simulink model "quadrotor"  (R2018b)
settings: Solver=VariableStepAuto  StartTime=0.0  StopTime=30  MaxStep=1e-1  RelTol=1e-3  EnableMultiTasking=on
values from neighbouring files (symbols this model uses):
  b = 0.6    [setup.m]
  d = 0.3    [setup.m]
  g = 9.81    [setup.m]
  m = 1    [setup.m]
  M2B_INV = inv(M2B)    [setup.m]
  P_q = 6    [setup.m]
  P_w = 1    [setup.m]
undefined symbols (not defined in the file or in its folder): X, Y, Z
libraries: nesl_utility x18, sm_lib x17
settings Model: Creator=valeriiche  LastModifiedBy=valeriiche
settings DataIOCC: LimitDataPoints=on
settings OptimizationCC: LifeSpan=inf
settings DebuggingCC: AllowSymbolicDim=off  SFUnexpectedBacktrackingDiag=warning  SFNoUnconditionalDefaultTransitionDiag=warning  SFExecutionAtInitializationDiag=none
settings SFSimCC: SimUseLocalCustomCode=off
settings RTWCC: RTWUseLocalCustomCode=off
settings CodeAppCC: StateflowObjectComments=on
settings GRTTargetCC: TargetLangStandard=C89/C90 (ANSI)  GeneratePreprocessorConditionals=Disable all
settings ConfigComp: CovMetricSettings=dw  CovHtmlReporting=on  CovSaveCumulativeToWorkspaceVar=on  CovSaveSingleToWorkspaceVar=on  CovExternalEMLEnable=off  CovSFcnEnable=off
settings SimscapeCC: SimscapeNominalValues="[{\"value\":\"10\",\"unit\":\"V\"},{\"value\":\"1\",\"unit\":\"A\"},{\"value\":\"10\",\"unit\":\"N*m\"},{\"value\":\"10\",\"unit\":\"bar\"},{\"value\":\"100\",\"unit\":\"kJ/kg\"},{\"value\":\"1\",\"unit\":\"kW\"},{\"value\":\"300\",\"unit\":\"K\"},{\"value\":\"100\",\"unit\":\"cm^3/s\"},{\"value\":\"1\",\"unit\":\"kN\"},{\"value\":\"1\",\"unit\":\"g/cm^3\"},{\"value\":\"1\",\"unit\":\"l\"},{\"value\":\"1\",\"unit\":\"cm^2\"},{\"value\":\"60\",\"unit\":\"Hz\"}]"  SimscapeLogType=all  SimscapeLogDataHistory=10000
settings ConfigurationSet: Description=SimMechanics 2G

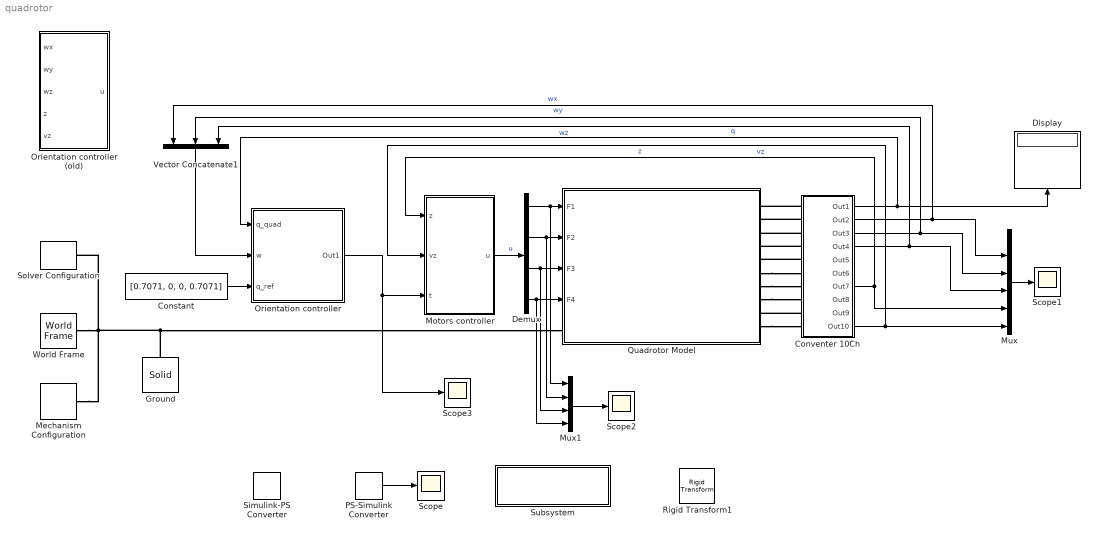
== system quadrotor ==
  Constant : Constant  Value=[0.7071, 0, 0, 0.7071]
  Conventer 10Ch : Subsystem
  Demux : Demux
  Display : Display
  Ground : sm_lib/Body Elements/Solid  InertiaType=CalculateFromGeometry  Mass=1  MassUnits=kg  CenterOfMass=[0 0 0]  CenterOfMassUnits=m  MomentsOfInertia=[1 1 1]  MomentsOfInertiaUnits=kg*m^2  ProductsOfInertia=[0 0 0]  ProductsOfInertiaUnits=kg*m^2  BasedOnType=Density  Density=1000  DensityUnits=kg/m^3  DoExposeReferenceFrame=on  SerializedFrames=<Frames/>  GraphicType=FromGeometry  MarkerShape=Sphere  MarkerSize=10  GraphicVisPropType=SimpleVisualProperties  GraphicDiffuseColor=[0.5 0.5 0.5]  GraphicSpecularColor=[0.5 0.5 0.5 1.0]  GraphicAmbientColor=[0.15 0.15 0.15 1.0]  GraphicEmissiveColor=[0.0 0.0 0.0 1.0]  GraphicShininess=75  GraphicOpacity=1.0  GeometryShape=Brick  RectangleSize=[1 1]  RectangleSizeUnits=m  BrickDimensions=[5 5 0.1]  BrickDimensionUnits=m  CylinderRadius=1  CylinderRadiusUnits=m  CylinderLength=1  CylinderLengthUnits=m  SphereRadius=1  SphereRadiusUnits=m  EllipsoidRadii=[1 1 1]  EllipsoidRadiiUnits=m  ExtrusionCrossSection=[1 1; -1 1; -1 -1; 1 -1]  ExtrusionCrossSectionUnits=m  ExtrusionLength=1  ExtrusionLengthUnits=m  PolygonNumSides=3  PolygonOuterRadius=1  PolygonOuterRadiusUnits=m  ExtGeomFileType=STEP  ExtGeomFileUnits=m  RevolutionCrossSection=[1 1; 1 -1; 2 -1; 2 1]  RevolutionCrossSectionUnits=m  RevolutionExtent=Full  RevolutionAngle=180  RevolutionAngleUnits=deg
  Mechanism Configuration : sm_lib/Utilities/Mechanism Configuration  UniformGravity=Constant  GravityVector=[0 0 -9.80665]  GravityUnits=m/s^2  LinearizationDelta=0.001
  Motors controller : Subsystem
  Mux : Mux  Inputs=6
  Mux1 : Mux
  Orientation controller : Subsystem
  Orientation controller (old) : Subsystem
  PS-Simulink Converter : nesl_utility/PS-Simulink Converter  PhysicalDomain=network_engine_domain  SubClassName=ps_output  LeftPortType=input  RightPortType=output  PseudoPeriodic=off  Frequencies=[]  Unit=1  AffineConversion=off
  Quadrotor Model : Subsystem
  Rigid Transform1 : sm_lib/Frames and Transforms/Rigid Transform  TranslationMethod=None  TranslationStandardOffset=0  TranslationLengthUnit=m  TranslationStandardAxis=+Z  TranslationCartesianOffset=[0 0 0]  TranslationROffset=0  TranslationROffsetUnits=m  TranslationZOffset=0  TranslationZOffsetUnits=m  TranslationThetaOffset=0  TranslationThetaOffsetUnits=deg  RotationMethod=None  RotationAngleUnits=deg  RotationStandardAxis=+Z  RotationAngle=0.0  RotationArbitraryAxis=[0 0 1]  FollAlignAxisA=+X  BaseAlignAxisA=+Y  FollAlignAxisB=+Y  BaseAlignAxisB=+Z  RotationSequenceAxes=FollowerAxes  RotationSequence=XYX  RotationSequenceAngles=[0 0 0]  RotationSequenceAnglesUnits=deg  RotationMatrix=[1 0 0; 0 1 0; 0 0 1]
  Scope{,1..3} (4 alike) : Scope
  Simulink-PS Converter : nesl_utility/Simulink-PS Converter  PhysicalDomain=network_engine_domain  SubClassName=ps_input  LeftPortType=input  RightPortType=output  PseudoPeriodic=off  Frequencies=[]  NoiseDistribution=none  NoiseParameters=[]  Unit=1  AffineConversion=off  FilteringAndDerivatives=zero  SimscapeFilterOrder=1  InputFilterTimeConstant=0.001  UdotUserProvided=1
  Solver Configuration : nesl_utility/Solver Configuration  PhysicalDomain=network_engine_domain  SubClassName=solver  LeftPortType=input  RightPortType=generic  Tones=[]  Harmonics=[]  SimulateNoise=off  Profile=off  UseLocalSampling=off  EnableSwitchedLinearOptims=on  FrequencyDomain=off  UseCCode=off  RelTol=0.001  AbsTol=1e-06  MinStep=1e-09  ToWorkspace=off  RevertToSquareIcSolve=off  NumHomotopyIterations=100  PhasorMode=off  PhasorModeNumHarmonics=1  DoDC=off  ResidualTolerance=1e-09  UseLocalSolver=off  LocalSolverChoice=NE_BACKWARD_EULER_ADVANCER  LocalSolverSampleTime=0.001  DoFixedCost=off  MaxNonlinIter=3  MaxModeIter=2  LinearAlgebra=Sparse  EquationFormulation=NE_TIME_EF  DelaysMemoryBudget=1024  AutomaticFiltering=on  FilteringTimeConstant=0.001  PartitionStorageMethod=AS_NEEDED  PartitionMemoryBudget=1024
  Subsystem : Subsystem
      settings: OpenFcn=open_system('sm_lib')
      mask Display: disp(sprintf('Open Simscape Multibody\nLibrary'));
  Vector Concatenate1 : Concatenate  NumInputs=3
  World Frame : sm_lib/Frames and Transforms/World Frame
  wires:
  PS-Simulink Converter/1 -> Scope/1
  Mux/1 -> Scope1/1
  Conventer 10Ch/3(Out3) -> Mux/3, Vector Concatenate1/2  "wy"
  Conventer 10Ch/7(Out7) -> Mux/5, Motors controller/1(z)  "z"
  Conventer 10Ch/10(Out10) -> Mux/6, Motors controller/2(vz)  "vz"
  Conventer 10Ch/4(Out4) -> Mux/4, Vector Concatenate1/3  "wz"
  Conventer 10Ch/2(Out2) -> Mux/2, Vector Concatenate1/1  "wx"
  Demux/1 -> Mux1/1, Quadrotor Model/1(F1)
  Demux/2 -> Mux1/2, Quadrotor Model/2(F2)
  Conventer 10Ch/1(Out1) -> Orientation controller/1(q_quad), Display/1  "q"
  Motors controller/1(u) -> Demux/1  "u"
  Orientation controller/1(Out1) -> Scope3/1, Motors controller/3(t)
  Vector Concatenate1/1 -> Orientation controller/2(w)
  Constant/1 -> Orientation controller/3(q_ref)
  Mux1/1 -> Scope2/1
  Demux/3 -> Mux1/3, Quadrotor Model/3(F3)
  Demux/4 -> Mux1/4, Quadrotor Model/4(F4)
  connections:
  Ground/RConn1 -- Quadrotor Model/LConn1 -- Solver Configuration/RConn1 -- Mechanism Configuration/RConn1 -- World Frame/RConn1
  Conventer 10Ch/LConn1 -- Quadrotor Model/RConn1
  Conventer 10Ch/LConn2 -- Quadrotor Model/RConn2
  Conventer 10Ch/LConn3 -- Quadrotor Model/RConn3
  Conventer 10Ch/LConn4 -- Quadrotor Model/RConn4
  Conventer 10Ch/LConn5 -- Quadrotor Model/RConn5
  Quadrotor Model/RConn6 -- Conventer 10Ch/LConn6
  Quadrotor Model/RConn7 -- Conventer 10Ch/LConn7
  Quadrotor Model/RConn8 -- Conventer 10Ch/LConn8
  Conventer 10Ch/LConn9 -- Quadrotor Model/RConn9
  Quadrotor Model/RConn10 -- Conventer 10Ch/LConn10

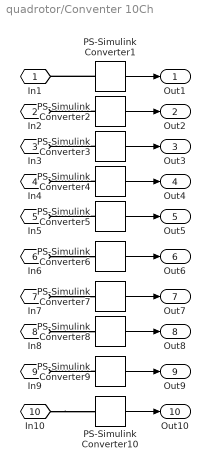
== system quadrotor/Conventer 10Ch ==
  PS-Simulink Converter{1..10} (10 alike) : nesl_utility/PS-Simulink Converter  PhysicalDomain=network_engine_domain  SubClassName=ps_output  LeftPortType=input  RightPortType=output  PseudoPeriodic=off  Frequencies=[]  Unit=1  AffineConversion=off
  In1 : PMIOPort  Side=Left
  In2 : PMIOPort  Port=2  Side=Left
  In3 : PMIOPort  Port=3  Side=Left
  In4 : PMIOPort  Port=4  Side=Left
  In5 : PMIOPort  Port=5  Side=Left
  In6 : PMIOPort  Port=6  Side=Left
  In7 : PMIOPort  Port=7  Side=Left
  In8 : PMIOPort  Port=8  Side=Left
  In9 : PMIOPort  Port=9  Side=Left
  In10 : PMIOPort  Port=10  Side=Left
  Out1 : Outport
  Out2 : Outport  Port=2
  Out3 : Outport  Port=3
  Out4 : Outport  Port=4
  Out5 : Outport  Port=5
  Out6 : Outport  Port=6
  Out7 : Outport  Port=7
  Out8 : Outport  Port=8
  Out9 : Outport  Port=9
  Out10 : Outport  Port=10
  wires:
  PS-Simulink Converter7/1 -> Out7/1
  PS-Simulink Converter4/1 -> Out4/1
  PS-Simulink Converter6/1 -> Out6/1
  PS-Simulink Converter8/1 -> Out8/1
  PS-Simulink Converter5/1 -> Out5/1
  PS-Simulink Converter9/1 -> Out9/1
  PS-Simulink Converter10/1 -> Out10/1
  PS-Simulink Converter3/1 -> Out3/1
  PS-Simulink Converter1/1 -> Out1/1
  PS-Simulink Converter2/1 -> Out2/1
  connections:
  In7/RConn1 -- PS-Simulink Converter7/LConn1
  PS-Simulink Converter1/LConn1 -- In1/RConn1
  PS-Simulink Converter3/LConn1 -- In3/RConn1
  In10/RConn1 -- PS-Simulink Converter10/LConn1
  PS-Simulink Converter2/LConn1 -- In2/RConn1
  In6/RConn1 -- PS-Simulink Converter6/LConn1
  PS-Simulink Converter5/LConn1 -- In5/RConn1
  PS-Simulink Converter4/LConn1 -- In4/RConn1
  In8/RConn1 -- PS-Simulink Converter8/LConn1
  PS-Simulink Converter9/LConn1 -- In9/RConn1

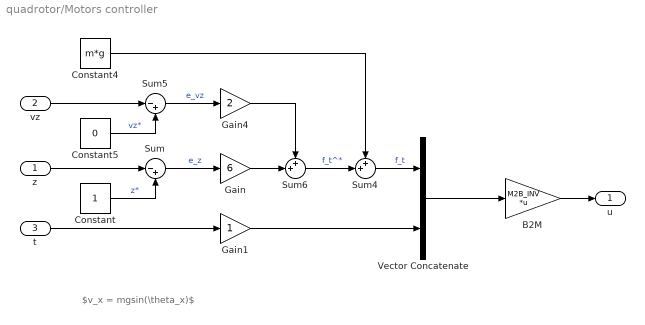
== system quadrotor/Motors controller ==
  note: $v_x = mgsin(\theta_x)$
  z : Inport
  vz : Inport  Port=2
  t : Inport  Port=3
  B2M : Gain  Gain=M2B_INV  Multiplication=Matrix(K*u) (u vector)
  Constant : Constant
  Constant4 : Constant  Value=m*g
  Constant5 : Constant  Value=0
  Gain : Gain  Gain=6
  Gain1 : Gain
  Gain4 : Gain  Gain=2
  Sum : Sum  Inputs=|-+
  Sum4 : Sum  Inputs=++|
  Sum5 : Sum  Inputs=|-+
  Sum6 : Sum  Inputs=++|
  Vector Concatenate : Concatenate
  u : Outport
  wires:
  Sum5/1 -> Gain4/1  "e_vz"
  B2M/1 -> u/1
  Gain/1 -> Sum6/2
  Gain4/1 -> Sum6/1
  z/1 -> Sum/1
  Sum4/1 -> Vector Concatenate/1  "f_t"
  Sum6/1 -> Sum4/2  "f_t^*"
  t/1 -> Gain1/1
  Constant5/1 -> Sum5/2  "vz*"
  Sum/1 -> Gain/1  "e_z"
  Vector Concatenate/1 -> B2M/1
  Gain1/1 -> Vector Concatenate/2
  Constant/1 -> Sum/2  "z*"
  Constant4/1 -> Sum4/1
  vz/1 -> Sum5/1

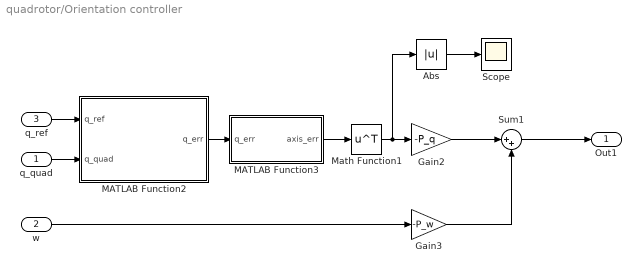
== system quadrotor/Orientation controller ==
  q_quad : Inport
  w : Inport  Port=2
  q_ref : Inport  Port=3
  Abs : Abs
  Gain2 : Gain  Gain=-P_q
  Gain3 : Gain  Gain=-P_w
  MATLAB Function2 : MATLAB Function  TreatAsAtomicUnit=on
  MATLAB Function3 : MATLAB Function  TreatAsAtomicUnit=on
  Math Function1 : Math  Operator=transpose  SaturateOnIntegerOverflow=on
  Scope : Scope
  Sum1 : Sum  Inputs=|++
  Out1 : Outport
  wires:
  Sum1/1 -> Out1/1
  Math Function1/1 -> Abs/1, Gain2/1
  MATLAB Function2/1(q_err) -> MATLAB Function3/1(q_err)
  Gain2/1 -> Sum1/1
  MATLAB Function3/1(axis_err) -> Math Function1/1
  Gain3/1 -> Sum1/2
  q_quad/1 -> MATLAB Function2/2(q_quad)
  q_ref/1 -> MATLAB Function2/1(q_ref)
  w/1 -> Gain3/1
  Abs/1 -> Scope/1

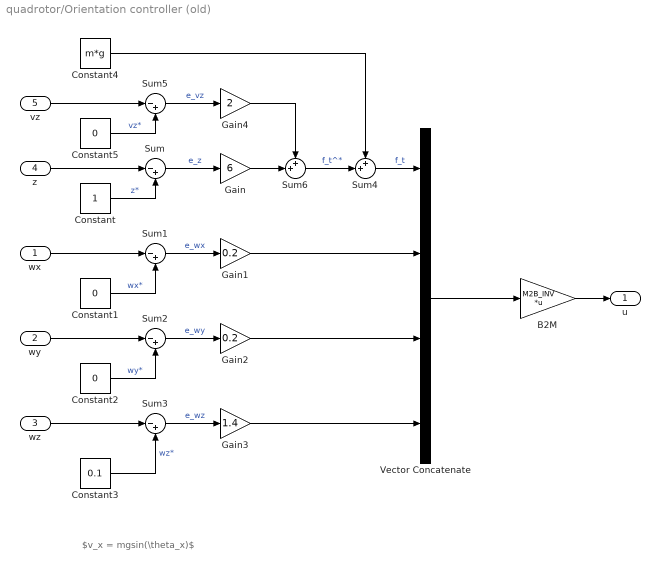
== system quadrotor/Orientation controller (old) ==
  note: $v_x = mgsin(\theta_x)$
  wx : Inport
  wy : Inport  Port=2
  wz : Inport  Port=3
  z : Inport  Port=4
  vz : Inport  Port=5
  B2M : Gain  Gain=M2B_INV  Multiplication=Matrix(K*u) (u vector)
  Constant : Constant
  Constant1 : Constant  Value=0
  Constant2 : Constant  Value=0
  Constant3 : Constant  Value=0.1
  Constant4 : Constant  Value=m*g
  Constant5 : Constant  Value=0
  Gain : Gain  Gain=6
  Gain1 : Gain  Gain=0.2
  Gain2 : Gain  Gain=0.2
  Gain3 : Gain  Gain=1.4
  Gain4 : Gain  Gain=2
  Sum{,1..3,5} (5 alike) : Sum  Inputs=|-+
  Sum4 : Sum  Inputs=++|
  Sum6 : Sum  Inputs=++|
  Vector Concatenate : Concatenate  NumInputs=4
  u : Outport
  wires:
  vz/1 -> Sum5/1
  Constant3/1 -> Sum3/2  "wz*"
  wx/1 -> Sum1/1
  Constant4/1 -> Sum4/1
  Constant/1 -> Sum/2  "z*"
  Sum3/1 -> Gain3/1  "e_wz"
  Gain1/1 -> Vector Concatenate/2
  Vector Concatenate/1 -> B2M/1
  Gain3/1 -> Vector Concatenate/4
  Sum/1 -> Gain/1  "e_z"
  wy/1 -> Sum2/1
  Constant2/1 -> Sum2/2  "wy*"
  Constant1/1 -> Sum1/2  "wx*"
  Sum2/1 -> Gain2/1  "e_wy"
  Constant5/1 -> Sum5/2  "vz*"
  Sum1/1 -> Gain1/1  "e_wx"
  wz/1 -> Sum3/1
  Sum6/1 -> Sum4/2  "f_t^*"
  Sum4/1 -> Vector Concatenate/1  "f_t"
  z/1 -> Sum/1
  Gain4/1 -> Sum6/1
  Gain2/1 -> Vector Concatenate/3
  Gain/1 -> Sum6/2
  B2M/1 -> u/1
  Sum5/1 -> Gain4/1  "e_vz"

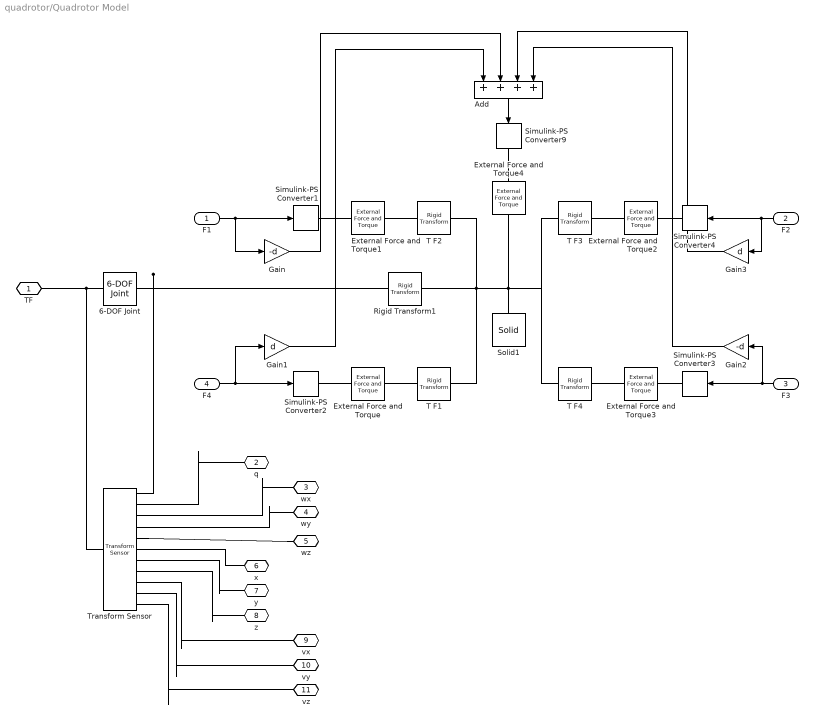
== system quadrotor/Quadrotor Model ==
  F1 : Inport
  F2 : Inport  Port=2
  F3 : Inport  Port=3
  F4 : Inport  Port=4
  6-DOF Joint : sm_lib/Joints/6-DOF Joint  SenseConstraintForce=off  SenseConstraintForceX=off  SenseConstraintForceY=off  SenseConstraintForceZ=off  SenseConstraintTorque=off  SenseConstraintTorqueX=off  SenseConstraintTorqueY=off  SenseConstraintTorqueZ=off  SenseTotalForce=off  SenseTotalForceX=off  SenseTotalForceY=off  SenseTotalForceZ=off  SenseTotalTorque=off  SenseTotalTorqueX=off  SenseTotalTorqueY=off  SenseTotalTorqueZ=off  CompositeWrenchDir=FollowerOnBase  CompositeWrenchFrame=BaseFrame  PxEquilibriumPosition=0  PxEquilibriumPositionUnits=m  PxSpringStiffness=0  PxSpringStiffnessUnits=N/m  PxDampingCoefficient=0  PxDampingCoefficientUnits=N/(m/s)  PxTorqueActuationMode=NoTorque  PxMotionActuationMode=ComputedMotion  PxSensePosition=off  PxSenseVelocity=off  PxSenseAcceleration=off  PxSenseTorqueForce=off  PxPositionTargetSpecify=off  PxPositionTargetPriority=High  PxPositionTargetValue=0  PxPositionTargetValueUnits=m  PxVelocityTargetSpecify=off  PxVelocityTargetPriority=High  PxVelocityTargetValue=0  PxVelocityTargetValueUnits=m/s  PyEquilibriumPosition=0  PyEquilibriumPositionUnits=m  PySpringStiffness=0  PySpringStiffnessUnits=N/m  PyDampingCoefficient=0  PyDampingCoefficientUnits=N/(m/s)  PyTorqueActuationMode=NoTorque  PyMotionActuationMode=ComputedMotion  PySensePosition=off  PySenseVelocity=off  PySenseAcceleration=off  PySenseTorqueForce=off  PyPositionTargetSpecify=off  PyPositionTargetPriority=High  PyPositionTargetValue=0  PyPositionTargetValueUnits=m  PyVelocityTargetSpecify=off  PyVelocityTargetPriority=High  PyVelocityTargetValue=0  PyVelocityTargetValueUnits=m/s  PzEquilibriumPosition=0  PzEquilibriumPositionUnits=m  PzSpringStiffness=0  PzSpringStiffnessUnits=N/m  PzDampingCoefficient=0  PzDampingCoefficientUnits=N/(m/s)  PzTorqueActuationMode=NoTorque  PzMotionActuationMode=ComputedMotion  PzSensePosition=off  PzSenseVelocity=off  PzSenseAcceleration=off  PzSenseTorqueForce=off  PzPositionTargetSpecify=on  PzPositionTargetPriority=Low  PzPositionTargetValue=b/5  PzPositionTargetValueUnits=m  PzVelocityTargetSpecify=off  PzVelocityTargetPriority=High  PzVelocityTargetValue=0  PzVelocityTargetValueUnits=m/s  SphDefPosRotationMethod=None  SphDefPosRotationAngleUnits=deg  SphDefPosRotationStandardAxis=+Z  SphDefPosRotationAngle=0.0  SphDefPosRotationArbitraryAxis=[0 0 1]  SphDefPosFollAlignAxisA=+X  SphDefPosBaseAlignAxisA=+Y  SphDefPosFollAlignAxisB=+Y  SphDefPosBaseAlignAxisB=+Z  SphDefPosRotationSequenceAxes=FollowerAxes  SphDefPosRotationSequence=XYX  SphDefPosRotationSequenceAngles=[0 0 0]  SphDefPosRotationSequenceAnglesUnits=deg  SphDefPosRotationMatrix=[1 0 0; 0 1 0; 0 0 1]  SphEqPosRotationMethod=None  SphEqPosRotationAngleUnits=deg  SphEqPosRotationStandardAxis=+Z  SphEqPosRotationAngle=0.0  SphEqPosRotationArbitraryAxis=[0 0 1]  SphEqPosFollAlignAxisA=+X  SphEqPosBaseAlignAxisA=+Y  SphEqPosFollAlignAxisB=+Y  SphEqPosBaseAlignAxisB=+Z  SphEqPosRotationSequenceAxes=FollowerAxes  SphEqPosRotationSequence=XYX  SphEqPosRotationSequenceAngles=[0 0 0]  SphEqPosRotationSequenceAnglesUnits=deg  SphEqPosRotationMatrix=[1 0 0; 0 1 0; 0 0 1]  SphSpringStiffness=0  SphSpringStiffnessUnits=N*m/deg  SphDampingCoefficient=0  SphDampingCoefficientUnits=N*m/(deg/s)  SphActuateTorqueX=off  SphActuateTorqueY=off  SphActuateTorqueZ=off  SphActuateTorque=off  SphTorqueActuationMode=NoTorque  SphMotionActuationMode=ComputedMotion  SphActuationFrame=BaseFrame  SphSensePosition=off  SphSenseVelocityX=off  SphSenseVelocityY=off  SphSenseVelocityZ=off  SphSenseVelocity=off  SphSenseAccelerationX=off  SphSenseAccelerationY=off  SphSenseAccelerationZ=off  SphSenseAcceleration=off  SphSenseTorqueX=off  SphSenseTorqueY=off  SphSenseTorqueZ=off  SphSenseTorqueForce=off  SphSensingFrame=BaseFrame  SphPositionTargetRotationMethod=None  SphPositionTargetRotationAngleUnits=deg  SphPositionTargetRotationStandardAxis=+Z  SphPositionTargetRotationAngle=0.0  SphPositionTargetRotationArbitraryAxis=[0 0 1]  SphPositionTargetFollAlignAxisA=+X  SphPositionTargetBaseAlignAxisA=+Y  SphPositionTargetFollAlignAxisB=+Y  SphPositionTargetBaseAlignAxisB=+Z  SphPositionTargetRotationSequenceAxes=FollowerAxes  SphPositionTargetRotationSequence=XYX  SphPositionTargetRotationSequenceAngles=[0 0 0]  SphPositionTargetRotationSequenceAnglesUnits=deg  SphPositionTargetRotationMatrix=[1 0 0; 0 1 0; 0 0 1]  SphPositionTargetSpecify=off  SphPositionTargetPriority=High  SphVelocityTargetValue=[0 0 0]  SphVelocityTargetValueUnits=deg/s  SphVelocityTargetSpecify=off  SphVelocityTargetPriority=High  SphVelocityTargetInFollowerFrame=on
  Add : Sum  Inputs=++++
  External Force and Torque{,1..3} (4 alike) : sm_lib/Forces and Torques/External Force and Torque  ForceResolutionFrame=AttachedFrame  EnableForceX=off  EnableForceY=off  EnableForceZ=on  EnableForce=off  TorqueResolutionFrame=AttachedFrame  EnableTorqueX=off  EnableTorqueY=off  EnableTorqueZ=off  EnableTorque=off
  External Force and Torque4 : sm_lib/Forces and Torques/External Force and Torque  ForceResolutionFrame=AttachedFrame  EnableForceX=off  EnableForceY=off  EnableForceZ=off  EnableForce=off  TorqueResolutionFrame=AttachedFrame  EnableTorqueX=off  EnableTorqueY=off  EnableTorqueZ=on  EnableTorque=off
  Gain : Gain  Gain=-d
  Gain1 : Gain  Gain=d
  Gain2 : Gain  Gain=-d
  Gain3 : Gain  Gain=d
  Rigid Transform1 : sm_lib/Frames and Transforms/Rigid Transform  TranslationMethod=None  TranslationStandardOffset=0  TranslationLengthUnit=m  TranslationStandardAxis=+Z  TranslationCartesianOffset=[-b/2 -b/2 0]  TranslationROffset=0  TranslationROffsetUnits=m  TranslationZOffset=0  TranslationZOffsetUnits=m  TranslationThetaOffset=0  TranslationThetaOffsetUnits=deg  RotationMethod=StandardAxis  RotationAngleUnits=deg  RotationStandardAxis=+Z  RotationAngle=45.0  RotationArbitraryAxis=[0 0 1]  FollAlignAxisA=+X  BaseAlignAxisA=+Y  FollAlignAxisB=+Y  BaseAlignAxisB=+Z  RotationSequenceAxes=FollowerAxes  RotationSequence=XYX  RotationSequenceAngles=[0 0 0]  RotationSequenceAnglesUnits=deg  RotationMatrix=[1 0 0; 0 1 0; 0 0 1]
  Simulink-PS Converter{1..4,9} (5 alike) : nesl_utility/Simulink-PS Converter  PhysicalDomain=network_engine_domain  SubClassName=ps_input  LeftPortType=input  RightPortType=output  PseudoPeriodic=off  Frequencies=[]  NoiseDistribution=none  NoiseParameters=[]  Unit=1  AffineConversion=off  FilteringAndDerivatives=zero  SimscapeFilterOrder=1  InputFilterTimeConstant=0.001  UdotUserProvided=1
  Solid1 : sm_lib/Body Elements/Solid  InertiaType=Custom  Mass=m  MassUnits=kg  CenterOfMass=[0 0 0]  CenterOfMassUnits=m  MomentsOfInertia=[1 1 1]  MomentsOfInertiaUnits=kg*m^2  ProductsOfInertia=[0 0 0]  ProductsOfInertiaUnits=kg*m^2  BasedOnType=Density  Density=1000  DensityUnits=kg/m^3  DoExposeReferenceFrame=on  SerializedFrames=<Frames/>  GraphicType=FromGeometry  MarkerShape=Sphere  MarkerSize=10  GraphicVisPropType=SimpleVisualProperties  GraphicDiffuseColor=[0.2 0.6 1.0]  GraphicSpecularColor=[0.5 0.5 0.5 1.0]  GraphicAmbientColor=[0.15 0.15 0.15 1.0]  GraphicEmissiveColor=[0.0 0.0 0.0 1.0]  GraphicShininess=75  GraphicOpacity=1.0  GeometryShape=Brick  RectangleSize=[1 1]  RectangleSizeUnits=m  BrickDimensions=[b b b/5]  BrickDimensionUnits=m  CylinderRadius=1  CylinderRadiusUnits=m  CylinderLength=1  CylinderLengthUnits=m  SphereRadius=1  SphereRadiusUnits=m  EllipsoidRadii=[1 1 1]  EllipsoidRadiiUnits=m  ExtrusionCrossSection=[1 1; -1 1; -1 -1; 1 -1]  ExtrusionCrossSectionUnits=m  ExtrusionLength=1  ExtrusionLengthUnits=m  PolygonNumSides=3  PolygonOuterRadius=1  PolygonOuterRadiusUnits=m  ExtGeomFileType=STEP  ExtGeomFileUnits=m  RevolutionCrossSection=[1 1; 1 -1; 2 -1; 2 1]  RevolutionCrossSectionUnits=m  RevolutionExtent=Full  RevolutionAngle=180  RevolutionAngleUnits=deg
  T F1 : sm_lib/Frames and Transforms/Rigid Transform  TranslationMethod=Cartesian  TranslationStandardOffset=0  TranslationLengthUnit=m  TranslationStandardAxis=+Z  TranslationCartesianOffset=[-b/2 b/2 0]  TranslationROffset=0  TranslationROffsetUnits=m  TranslationZOffset=0  TranslationZOffsetUnits=m  TranslationThetaOffset=0  TranslationThetaOffsetUnits=deg  RotationMethod=None  RotationAngleUnits=deg  RotationStandardAxis=+Z  RotationAngle=0.0  RotationArbitraryAxis=[0 0 1]  FollAlignAxisA=+X  BaseAlignAxisA=+Y  FollAlignAxisB=+Y  BaseAlignAxisB=+Z  RotationSequenceAxes=FollowerAxes  RotationSequence=XYX  RotationSequenceAngles=[0 0 0]  RotationSequenceAnglesUnits=deg  RotationMatrix=[1 0 0; 0 1 0; 0 0 1]
  T F2 : sm_lib/Frames and Transforms/Rigid Transform  TranslationMethod=Cartesian  TranslationStandardOffset=0  TranslationLengthUnit=m  TranslationStandardAxis=+Z  TranslationCartesianOffset=[b/2 b/2 0]  TranslationROffset=0  TranslationROffsetUnits=m  TranslationZOffset=0  TranslationZOffsetUnits=m  TranslationThetaOffset=0  TranslationThetaOffsetUnits=deg  RotationMethod=None  RotationAngleUnits=deg  RotationStandardAxis=+Z  RotationAngle=0.0  RotationArbitraryAxis=[0 0 1]  FollAlignAxisA=+X  BaseAlignAxisA=+Y  FollAlignAxisB=+Y  BaseAlignAxisB=+Z  RotationSequenceAxes=FollowerAxes  RotationSequence=XYX  RotationSequenceAngles=[0 0 0]  RotationSequenceAnglesUnits=deg  RotationMatrix=[1 0 0; 0 1 0; 0 0 1]
  T F3 : sm_lib/Frames and Transforms/Rigid Transform  TranslationMethod=Cartesian  TranslationStandardOffset=0  TranslationLengthUnit=m  TranslationStandardAxis=+Z  TranslationCartesianOffset=[b/2 -b/2 0]  TranslationROffset=0  TranslationROffsetUnits=m  TranslationZOffset=0  TranslationZOffsetUnits=m  TranslationThetaOffset=0  TranslationThetaOffsetUnits=deg  RotationMethod=None  RotationAngleUnits=deg  RotationStandardAxis=+Z  RotationAngle=0.0  RotationArbitraryAxis=[0 0 1]  FollAlignAxisA=+X  BaseAlignAxisA=+Y  FollAlignAxisB=+Y  BaseAlignAxisB=+Z  RotationSequenceAxes=FollowerAxes  RotationSequence=XYX  RotationSequenceAngles=[0 0 0]  RotationSequenceAnglesUnits=deg  RotationMatrix=[1 0 0; 0 1 0; 0 0 1]
  T F4 : sm_lib/Frames and Transforms/Rigid Transform  TranslationMethod=Cartesian  TranslationStandardOffset=0  TranslationLengthUnit=m  TranslationStandardAxis=+Z  TranslationCartesianOffset=[-b/2 -b/2 0]  TranslationROffset=0  TranslationROffsetUnits=m  TranslationZOffset=0  TranslationZOffsetUnits=m  TranslationThetaOffset=0  TranslationThetaOffsetUnits=deg  RotationMethod=None  RotationAngleUnits=deg  RotationStandardAxis=+Z  RotationAngle=0.0  RotationArbitraryAxis=[0 0 1]  FollAlignAxisA=+X  BaseAlignAxisA=+Y  FollAlignAxisB=+Y  BaseAlignAxisB=+Z  RotationSequenceAxes=FollowerAxes  RotationSequence=XYX  RotationSequenceAngles=[0 0 0]  RotationSequenceAnglesUnits=deg  RotationMatrix=[1 0 0; 0 1 0; 0 0 1]
  Transform Sensor : sm_lib/Frames and Transforms/Transform Sensor  MeasurementFrame=World  SenseAngle=off  SenseAxis=off  SenseAngle1=off  SenseAngle2=off  SenseAngle3=off  SenseQ=on  SenseR=off  SenseOmegaX=on  SenseOmegaY=on  SenseOmegaZ=on  SenseOmega1=off  SenseOmega2=off  SenseOmega3=off  SenseQDot=off  SenseRDot=off  SenseAlphaX=off  SenseAlphaY=off  SenseAlphaZ=off  SenseAlpha1=off  SenseAlpha2=off  SenseAlpha3=off  SenseQDDot=off  SenseRDDot=off  SenseX=on  SenseY=on  SenseZ=on  SenseRad=off  SenseAzim=off  SenseDist=off  SenseInc=off  SenseXDot=on  SenseYDot=on  SenseZDot=on  SenseRadDot=off  SenseAzimDot=off  SenseDistDot=off  SenseIncDot=off  SenseXDDot=off  SenseYDDot=off  SenseZDDot=off  SenseRadDDot=off  SenseAzimDDot=off  SenseDistDDot=off  SenseIncDDot=off
  TF : PMIOPort  Side=Left
  q : PMIOPort  Port=2  Side=Right
  wx : PMIOPort  Port=3  Side=Right
  wy : PMIOPort  Port=4  Side=Right
  wz : PMIOPort  Port=5  Side=Right
  x : PMIOPort  Port=6  Side=Right
  y : PMIOPort  Port=7  Side=Right
  z : PMIOPort  Port=8  Side=Right
  vx : PMIOPort  Port=9  Side=Right
  vy : PMIOPort  Port=10  Side=Right
  vz : PMIOPort  Port=11  Side=Right
  wires:
  F1/1 -> Gain/1, Simulink-PS Converter1/1
  F2/1 -> Gain3/1, Simulink-PS Converter4/1
  F4/1 -> Gain1/1, Simulink-PS Converter2/1
  Gain/1 -> Add/2
  Gain1/1 -> Add/1
  Gain2/1 -> Add/4
  F3/1 -> Gain2/1, Simulink-PS Converter3/1
  Add/1 -> Simulink-PS Converter9/1
  Gain3/1 -> Add/3
  connections:
  Transform Sensor/RConn10 -- vy/RConn1
  Simulink-PS Converter4/RConn1 -- External Force and Torque2/LConn1
  Transform Sensor/RConn3 -- wx/RConn1
  Transform Sensor/RConn8 -- z/RConn1
  Transform Sensor/RConn6 -- x/RConn1
  Simulink-PS Converter3/RConn1 -- External Force and Torque3/LConn1
  Transform Sensor/RConn9 -- vx/RConn1
  Transform Sensor/RConn2 -- q/RConn1
  Transform Sensor/RConn11 -- vz/RConn1
  Simulink-PS Converter2/RConn1 -- External Force and Torque/LConn1
  Transform Sensor/RConn4 -- wy/RConn1
  Transform Sensor/RConn7 -- y/RConn1
  Simulink-PS Converter1/RConn1 -- External Force and Torque1/LConn1
  Transform Sensor/RConn5 -- wz/RConn1
  Transform Sensor/LConn1 -- TF/RConn1 -- 6-DOF Joint/LConn1
  Solid1/RConn1 -- Rigid Transform1/LConn1 -- T F1/LConn1 -- T F2/LConn1 -- External Force and Torque4/RConn1 -- T F3/LConn1 -- T F4/LConn1
  Transform Sensor/RConn1 -- Rigid Transform1/RConn1 -- 6-DOF Joint/RConn1
  T F2/RConn1 -- External Force and Torque1/RConn1
  T F4/RConn1 -- External Force and Torque3/RConn1
  T F3/RConn1 -- External Force and Torque2/RConn1
  T F1/RConn1 -- External Force and Torque/RConn1
  Simulink-PS Converter9/RConn1 -- External Force and Torque4/LConn1

== system quadrotor/Subsystem ==

== matlab function quadrotor/Orientation controller/MATLAB Function2 ==
  data: q_ref input; q_err output; q_quad input
function q_err = orient_err(q_ref, q_quad)

q_quad_conj = [ q_quad(1), -q_quad(2), -q_quad(3), -q_quad(4) ];


% Q(q_ref) * q_quad_conj
q_err = [[ q_ref(1), -q_ref(2), -q_ref(3), -q_ref(4)];
         [ q_ref(2),  q_ref(1), -q_ref(4),  q_ref(3)];
         [ q_ref(3),  q_ref(4),  q_ref(1), -q_ref(2)];
         [ q_ref(4), -q_ref(3),  q_ref(2),  q_ref(1)]] * q_quad_conj';

% y = quat_multiply(q_ref, quat_conjugate(q_quad));

== matlab function quadrotor/Orientation controller/MATLAB Function3 ==
  data: q_err input; axis_err output
function axis_err = fcn(q_err)

ans = [q_err(2), q_err(3), q_err(4)];

% if q_err(1) < 0
%     ans = [-q_err(2), -q_err(3), -q_err(4)];
% else
%     ans = [q_err(2), q_err(3), q_err(4)];
% end

axis_err = ans;
